simulink model "closed_loop"  (R2020b)
settings: Solver=VariableStepAuto  StartTime=0.0  StopTime=1000  RelTol=1e-3
values from neighbouring files (symbols this model uses):
  A = zeros(size(B'))    [parameters.m]
  Ad = sysd.A    [mpc.m]    (also in parameters.m)
  B = [repmat(eye(3),[1 4]) ... (first row only)    [parameters.m]
  Bd = sysd.B    [mpc.m]    (also in parameters.m)
  I = 4000*eye(3)    [parameters.m]
  K_steer = lqr(Ae,Be,Q,10)    [parameters.m]
  mass = 2000    [parameters.m]
  N = size(R,1)/nStates-1    [body_force_mpc.m]    (also in mpc.m; parameters.m = 10)
  Qf = 1e3*eye(6)    [parameters.m]
  Qu = cost_matrix(Qu,N)    [body_force_mpc.m]    (also in mpc.m; parameters.m = 1e-3*eye(3))
  Qx = blkdiag(cost_matrix(Qx,N-1),Qf)    [body_force_mpc.m]    (also in mpc.m = cost_matrix(Qx,N); parameters.m = eye(6))
  R = R(:)    [body_force_mpc.m]    (also in generate_reference.m = zeros(length(r_0),length(t)); mpc.m; parameters.m = cell2mat(arrayfun(r,tau,'UniformOutput',false)); reference_generator.m = R(:,1:super_sample_ratio:end))
  r_1 = [front_length;width/2;-height]    [parameters.m]
  radius = 0.4    [parameters.m]
  rear_length = 1.6    [parameters.m]
  T = 0.1    [mpc.m]    (also in parameters.m)
  turn_limit = deg2rad(30)    [parameters.m]
  v_0 = 10    [parameters.m]
  width = 2    [parameters.m]
libraries: autolibshared x5, vrlib x4
(part 4 of 4)

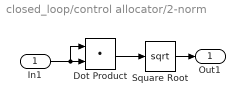
== system closed_loop/control allocator/2-norm ==
  In1 : Inport
  Dot Product : DotProduct  InputSameDT=on  OutDataTypeStr=Inherit: Inherit via internal rule
  Square Root : Sqrt  SaturateOnIntegerOverflow=on
  Out1 : Outport
  wires:
  Square Root/1 -> Out1/1
  Dot Product/1 -> Square Root/1
  In1/1 -> Dot Product/1, Dot Product/2

== system closed_loop/control allocator/2-norm1 ==
  In1 : Inport
  Dot Product : DotProduct  InputSameDT=on  OutDataTypeStr=Inherit: Inherit via internal rule
  Square Root : Sqrt  SaturateOnIntegerOverflow=on
  Out1 : Outport
  wires:
  Square Root/1 -> Out1/1
  Dot Product/1 -> Square Root/1
  In1/1 -> Dot Product/1, Dot Product/2

== system closed_loop/control allocator/2-norm2 ==
  In1 : Inport
  Dot Product : DotProduct  InputSameDT=on  OutDataTypeStr=Inherit: Inherit via internal rule
  Square Root : Sqrt  SaturateOnIntegerOverflow=on
  Out1 : Outport
  wires:
  Square Root/1 -> Out1/1
  Dot Product/1 -> Square Root/1
  In1/1 -> Dot Product/1, Dot Product/2

== system closed_loop/control allocator/2-norm3 ==
  In1 : Inport
  Dot Product : DotProduct  InputSameDT=on  OutDataTypeStr=Inherit: Inherit via internal rule
  Square Root : Sqrt  SaturateOnIntegerOverflow=on
  Out1 : Outport
  wires:
  Square Root/1 -> Out1/1
  Dot Product/1 -> Square Root/1
  In1/1 -> Dot Product/1, Dot Product/2

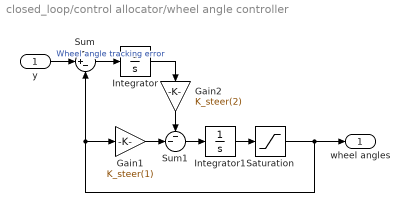
== system closed_loop/control allocator/wheel angle controller ==
  y : Inport
  Gain1 : Gain  Gain=K_steer(1)
  Gain2 : Gain  Gain=K_steer(2)
  Integrator : Integrator
  Integrator1 : Integrator
  Saturation : Saturate  UpperLimit=turn_limit  LowerLimit=-turn_limit
  Sum : Sum  Inputs=|+-
  Sum1 : Sum  Inputs=--|
  wheel angles : Outport
  wires:
  Sum/1 -> Integrator/1  "Wheel angle tracking error"
  y/1 -> Sum/1
  Integrator1/1 -> Saturation/1
  Saturation/1 -> wheel angles/1, Gain1/1, Sum/2
  Integrator/1 -> Gain2/1
  Sum1/1 -> Integrator1/1
  Gain1/1 -> Sum1/2
  Gain2/1 -> Sum1/1

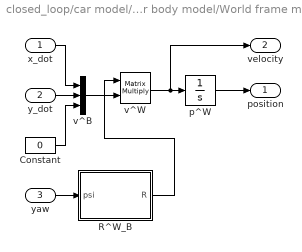
== system closed_loop/car model/car body model/World frame motion ==
  x_dot : Inport
  y_dot : Inport  Port=2
  yaw : Inport  Port=3
  Constant : Constant  Value=0
  R^W_B : MATLAB Function  TreatAsAtomicUnit=on
  p^W : Integrator
  v^B : Mux  Inputs=3
  v^W : Product  Multiplication=Matrix(*)
  position : Outport
  velocity : Outport  Port=2
  wires:
  yaw/1 -> R^W_B/1(psi)
  y_dot/1 -> v^B/2
  x_dot/1 -> v^B/1
  Constant/1 -> v^B/3
  v^B/1 -> v^W/2
  R^W_B/1(R) -> v^W/1
  v^W/1 -> velocity/1, p^W/1
  p^W/1 -> position/1

== matlab function closed_loop/control allocator/steering angles ==
  data: u input; y output
function y = modulo_forward(u)
min=-pi/2; max=pi/2;
y=mod(u-min,max-min)+min;

== matlab function closed_loop/allocator inverter/force_direction ==
  data: delta input; f output
function f = unit_vector(delta)
f=[cos(delta);sin(delta);0];

== matlab function closed_loop/allocator inverter/force_direction1 ==
  data: delta input; f output
function f = unit_vector(delta)
f=[cos(delta);sin(delta);0];

== matlab function closed_loop/allocator inverter/force_direction2 ==
  data: delta input; f output
function f = unit_vector(delta)
f=[cos(delta);sin(delta);0];

== matlab function closed_loop/allocator inverter/force_direction3 ==
  data: delta input; f output
function f = unit_vector(delta)
f=[cos(delta);sin(delta);0];

== matlab function closed_loop/model predictive controller/MATLAB Function ==
  settings: updateMethod=DISCRETE  sampleTime=T
  data: x input; u output; t input; N parameter; Qx parameter; Qu parameter; Qf parameter; Ad parameter; Bd parameter; T parameter; R parameter
function u=mpc(x,t,N, Qx, Qu, Qf, Ad, Bd, T, R)
    tau_0=round(t/T)+1;
    R=R(:,tau_0:min(tau_0+N,end));
    us=body_force_mpc(x,R,Qx,Qu,Qf,Ad,Bd);
    u=us(1:3,1);
end

== matlab function closed_loop/car model/longitudinal wheel motion/R^1_B ==
  data: delta input; R output
function R = wheel_rotation(delta)
R=[cos(delta) sin(delta) 0
  -sin(delta) cos(delta) 0
  0 0 1];

== matlab function closed_loop/car model/longitudinal wheel motion/R^2_B ==
  data: delta input; R output
function R = wheel_rotation(delta)
R=[cos(delta) sin(delta) 0
  -sin(delta) cos(delta) 0
  0 0 1];

== matlab function closed_loop/car model/longitudinal wheel motion/R^3_B ==
  data: delta input; R output
function R = wheel_rotation(delta)
R=[cos(delta) sin(delta) 0
  -sin(delta) cos(delta) 0
  0 0 1];

== matlab function closed_loop/car model/longitudinal wheel motion/R^4_B ==
  data: delta input; R output
function R = wheel_rotation(delta)
R=[cos(delta) sin(delta) 0
  -sin(delta) cos(delta) 0
  0 0 1];

== matlab function closed_loop/car model/car body model/World frame motion/R^W_B ==
  data: psi input; R output
function R = rotation_matrix(psi)
R = [cos(psi) -sin(psi) 0
     sin(psi)  cos(psi) 0
     0         0        1];
